simulink model "Vehicle_Control_CodeGen"  (R2024a)
settings: Solver=FixedStepAuto  StartTime=0.0  StopTime=10  RelTol=1e-3  EnableMultiTasking=on
undefined symbols (not defined in the file or in its folder): CAN, DiscIntNeverNeededParam, FD, Ion, Lithium
libraries: stmutilitieslib x28, simulink x21, stm32blockslib x10, canfdmsglib x6, dspstat3 x6, slpidlib x3, spsBatteryLib x2, spsControlledCurrentSourceLib x2, spsVoltageMeasurementLib x2, spspowerguiLib x2, stm32h7xxblockslib x2
(part 1 of 3)
settings Model: STM32="{\"FDCANWrite\":[{\"ID\":\"Vehicle_Control_CodeGen:2627\"},{\"ID\":\"Vehicle_Control_CodeGen:2628\"},{\"ID\":\"Vehicle_Control_CodeGen:2945\"},{\"ID\":\"Vehicle_Control_CodeGen:2946\"},{\"ID\":\"Vehicle_Control_CodeGen:2660\"},{\"ID\":\"Vehicle_Control_CodeGen:2661\"},{\"ID\":\"Vehicle_Control_CodeGen:3556\"},{\"ID\":\"Vehicle_Control_CodeGen:3558\"}],\"FDCANRead\":[{\"ID\":\"Vehicle_Control_CodeGen:2697\"},{\"ID\":\"Vehicle_Control_CodeGen:2816\"}],\"HardwareInterrupt\":[{\"ID\":\"Vehicle_Control_CodeGen:2909\"},{\"ID\":\"Vehicle_Control_CodeGen:2910\"}]}"  Creator=ezeki  LastModifiedBy=ezeki
settings SolverCC: PositivePriorityOrder=on  AutoInsertRateTranBlk=on
settings OptimizationCC: EnhancedBackFolding=on  PassReuseOutputArgsAs=Individual arguments  ZeroExternalMemoryAtStartup=off  ZeroInternalMemoryAtStartup=off  MaxStackSize=512  OptimizeBlockOrder=speed  DifferentSizesBufferReuse=on  OptimizationCustomize=off  EfficientTunableParamExpr=on
settings DebuggingCC: MultiTaskDSMMsg=none  ParameterTunabilityLossMsg=error
settings HardwareCC: ProdBitPerPointer=32  ProdBitPerSizeT=32  ProdBitPerPtrDiffT=32  ProdLargestAtomicInteger=Long  ProdLargestAtomicFloat=Double  ProdWordSize=32  ProdLongLongMode=on  ProdHWDeviceType=ARM Compatible->ARM Cortex-M
settings SFSimCC: MATLABDynamicMemAlloc=off
settings RTWCC: Description=Embedded Coder  SystemTargetFile=ert.tlc  HardwareBoard=STM32H7xx Based (Single-core)  TLCOptions="-aInlineSetEventsForThisBaseRateFcn=TLC_FALSE -aSuppressMultiTaskScheduler=TLC_FALSE  -aRateBasedStepFcn=0"  TemplateMakefile=ert_default_tmf  Toolchain=GNU Tools for ARM Embedded Processors
settings CodeAppCC: ForceParamTrailComments=on  IgnoreCustomStorageClasses=off  OperatorAnnotations=on  SimulinkDataObjDesc=on  SFDataObjDesc=on  InsertBlockDesc=on
settings ERTTargetCC: TargetLangStandard=C99 (ISO)  CodeReplacementLibrary=ARM Cortex-M  ExtModeTransport=3  ExtModeStaticAlloc=on  ExtModeStaticAllocSize=2048  ExtModeMexFile=ext_xcp  ExtModeIntrfLevel=Level2 - Open

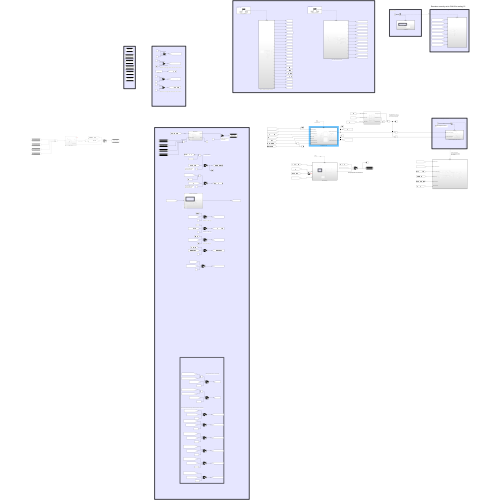
[thumbnail: Simulink's stored preview of the top-level diagram]
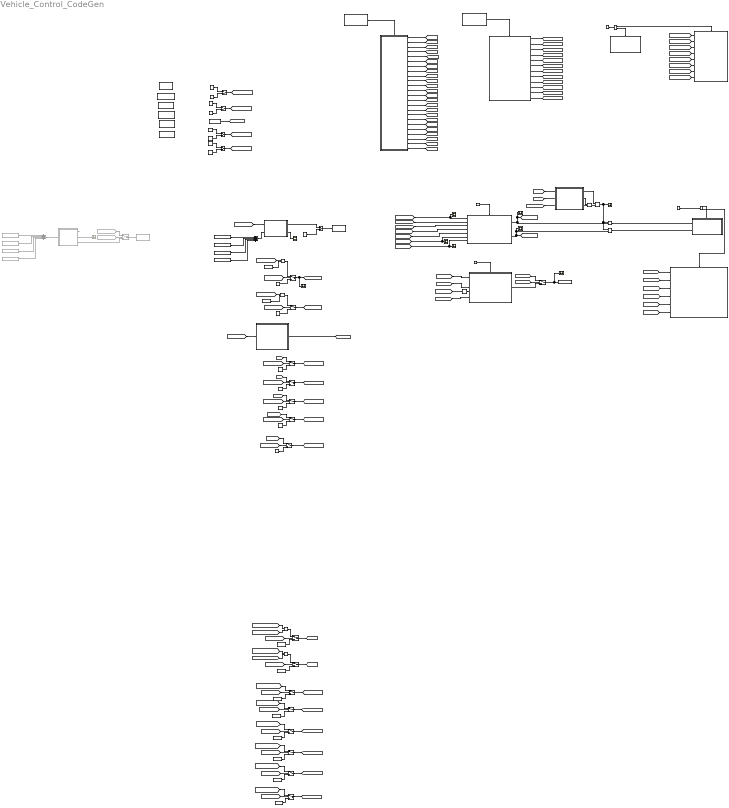
== system Vehicle_Control_CodeGen ==
  note: Because of the expected amount of acceleration between function call this function is also set to run at 50Hz.
  note: Derating values a scalers and are in the the magnitude of 0-1. The can be multiplied by with the requested power to scale them appropriatly.
  note: Takes the greater of the two for use in derating.
  note: Handy to test Can outputs. A constant can be put in to test transmission
  note: Greater then 5 enables regen
  note: Converts RPM to Rad/s
  note: PID Loop runs allot faster to minimise overshoot. Messages are sent at a slower rate.
  note: Remeber currently set to CAN 2 for testing !!!!
  note: Receiving Can messages from CAN 1 (front of vehicle) and Can 2 (inverters)
  note: These can also be used to test code gen. Shows that varibles are transmitting.
  note: Global Defines
  note: Set Max time to 2154 Length of dat set used for power control for endurance
  note: This Constant Can be changed to varible at a latter date for data playback/simulation
  note: All Global Varibles
  note: Simulation Varible Setup
  note: This can be configured for either endurance (Power Forcasting Used) Or other events (fixed power limit)
  note: Set to 500 Hz call
  note: This Constant Can be changed to varible at a latter date for data playback/simulation
  note: Set Max time to 2154 Length of dat set used for power control for endurance
  note: CAN 1 information from pedal box and dash.
  note: Inverter Can Setup
  note: CAN 2 Receive Data From Inverters
  note: Forwarding Messages From the Inverters to Data Logger
  note: Example On How to send Messages to Inverters
  note: Greater then 5 enables regen
  note: Less then 90 enables regen
  10 HZ Send1 : Subsystem  TreatAsAtomicUnit=on
  50 HZ Send Torque Requests to Inverters : Subsystem  TreatAsAtomicUnit=on
  Add : Sum  Commented=on  Inputs=++++
  Add1 : Sum  Inputs=++++
  Battery Model : Subsystem  Commented=on
  Constant{,5,14,24} (4 alike) : Constant
  Constant{1,6,8,15,25} (5 alike) : Constant  Value=0
  Constant{2,7,10..13} (6 alike) : Constant  Value=25000
  Constant16 : Constant  Value=0.10472
  Constant17 : Constant  Value=0.10472
  Constant18 : Constant  Value=6
  Constant19 : Constant  Value=85
  Constant20 : Constant  Value=580
  Constant21 : Constant  Value=20
  Constant22 : Constant  Value=40
  Constant23 : Constant  Value=60
  Constant3 : Constant  Value=10
  Constant4 : Constant  Value=10
  Constant9 : Constant  Value=6
  Data Store Memory : DataStoreMemory  DataStoreName=Battery_Voltage  WriteAfterWriteMsg=warning  ShowAdditionalParam=off
  Data Store Memory1 : DataStoreMemory  DataStoreName=Right_Sim_Discharge_Current  WriteAfterWriteMsg=warning  ShowAdditionalParam=off
  Data Store Memory2 : DataStoreMemory  DataStoreName=Right_Sim_Regen_Current  WriteAfterWriteMsg=warning  ShowAdditionalParam=off
  Data Store Memory3 : DataStoreMemory  DataStoreName=Left_Sim_Discharge_Current  WriteAfterWriteMsg=warning  ShowAdditionalParam=off
  Data Store Memory4 : DataStoreMemory  DataStoreName=Left_Sim_Regen_Current  WriteAfterWriteMsg=warning  ShowAdditionalParam=off
  Data Store Memory5 : DataStoreMemory  DataStoreName=Global_Power_Limit  WriteAfterWriteMsg=warning  ShowAdditionalParam=off
  Data Store Read : DataStoreRead  Commented=on  DataStoreName=Left_Sim_Discharge_Current  IndexOptions=Index vector (dialog)  Indices=1  OutputSizes=1
  Data Store Read1 : DataStoreRead  Commented=on  DataStoreName=Left_Sim_Regen_Current  IndexOptions=Index vector (dialog)  Indices=1  OutputSizes=1
  Data Store Read2 : DataStoreRead  Commented=on  DataStoreName=Right_Sim_Discharge_Current  IndexOptions=Index vector (dialog)  Indices=1  OutputSizes=1
  Data Store Read3 : DataStoreRead  Commented=on  DataStoreName=Right_Sim_Regen_Current  IndexOptions=Index vector (dialog)  Indices=1  OutputSizes=1
  Data Store Read4 : DataStoreRead  DataStoreName=Left_Sim_Discharge_Current  IndexOptions=Index vector (dialog)  Indices=1  OutputSizes=1
  Data Store Read5 : DataStoreRead  DataStoreName=Left_Sim_Regen_Current  IndexOptions=Index vector (dialog)  Indices=1  OutputSizes=1
  Data Store Read6 : DataStoreRead  DataStoreName=Right_Sim_Discharge_Current  IndexOptions=Index vector (dialog)  Indices=1  OutputSizes=1
  Data Store Read7 : DataStoreRead  DataStoreName=Right_Sim_Regen_Current  IndexOptions=Index vector (dialog)  Indices=1  OutputSizes=1
  Data Store Write : DataStoreWrite  Commented=on  DataStoreName=Battery_Voltage  IndexOptions=Index vector (dialog)  Indices=1  OutputSizes=1
  Data Store Write1 : DataStoreWrite  DataStoreName=Global_Power_Limit  IndexOptions=Index vector (dialog)  Indices=1  OutputSizes=1
  Data Store Write2 : DataStoreWrite  DataStoreName=Battery_Voltage  IndexOptions=Index vector (dialog)  Indices=1  OutputSizes=1
  From7 : From  Commented=on  GotoTag=Simulation_Enable
  From8 : From  Commented=on  GotoTag=CAN_Battery_Voltage
  Function-Call Generator : simulink/Ports & Subsystems/Function-Call Generator  sample_time=0.002  numberOfIterations=1  DisallowWideOutput=off
  Function-Call Generator1 : simulink/Ports & Subsystems/Function-Call Generator  sample_time=0.01  numberOfIterations=1  DisallowWideOutput=off
  Function-Call Generator2 : simulink/Ports & Subsystems/Function-Call Generator  sample_time=0.02  numberOfIterations=1  DisallowWideOutput=off
  Function-Call Generator4 : simulink/Ports & Subsystems/Function-Call Generator  sample_time=0.2  numberOfIterations=1  DisallowWideOutput=off
  Function-Call Split : FunctionCallSplit  IconShape=distinctive  NumOutputPorts=2  OutputPortLayout=default
  Function-Call Split1 : FunctionCallSplit  IconShape=distinctive  NumOutputPorts=2
  Function-Call Subsystem : Subsystem  TreatAsAtomicUnit=on
  Function-Call Subsystem1 : Subsystem  TreatAsAtomicUnit=on
  Hardware Interrupt1 : stm32h7xxblockslib/Hardware Interrupt  ISRGroup=Controller Area Network Flexible Data-Rate (FDCAN)  ISRName=FDCAN2_IT0_IRQHandler  ISRNumber=35  EventsList={ 'off', 'FDCAN2 HPME', '1'; 'off', 'FDCAN2 DRXE', '2'; 'on', 'FDCAN2 RF0NE', '3'; 'off', 'FDCAN2 RF0F', '4'; 'off', 'FDCAN2 RF0L', '5'; 'off', 'FDCAN2 RF0W', '6'; 'off', 'FDCAN2 RF1NE', '7'; 'off', 'FDCAN2 RF1F', '8'; 'off', 'FDCAN2 RF1L', '9'; 'off', 'FDCAN2 RF1W', '10'; 'off', 'FDCAN2 TC', '11'; 'off', 'FDCAN2 TCF', '12'; 'off', 'FDCAN2 TFE', '13'; 'off', 'FDCAN2 TEFN', '14'; 'off', 'FDCAN2 TEFL', '15'; 'off', 'FDCAN2 TEFF', '16'; 'off', 'FDCAN2 TEFW', '17'; 'off', 'FDCAN2 TSW', '18'; 'off', 'FDCAN2 MRAF', '19'; 'off', 'FDCAN2 TOO', '20'; 'off', 'FDCAN2 ELO', '21'; 'off', 'FDCAN2 EP', '22'; 'off', 'FDCAN2 EW', '23'; 'off', 'FDCAN2 BO', '24'; 'off', 'FDCAN2 WDI', '25'; 'off', 'FDCAN2 PEA', '26'; 'off', 'FDCAN2 PED', '27'; 'off', 'FDCAN2 ARA', '28'; 'off', 'Custom event', '29' }  SelectedEvents={'FDCAN2 RF0NE'}  TaskPriority=29  DisablePreemption=off  ClearInterruptFlagsAtEndOfEvent=off  InterruptDefinitionFile=$(TARGET_ROOT)/registry/interrupts/STM32F4xxBased_interrupts.xml  HardwareBoard=STM32H7xx Based  EnableSimPort=off
  Hardware Interrupt3 : stm32h7xxblockslib/Hardware Interrupt  ISRGroup=Controller Area Network Flexible Data-Rate (FDCAN)  ISRName=FDCAN1_IT0_IRQHandler  ISRNumber=34  EventsList={ 'off', 'FDCAN1 HPME', '1'; 'off', 'FDCAN1 DRXE', '2'; 'on', 'FDCAN1 RF0NE', '3'; 'off', 'FDCAN1 RF0F', '4'; 'off', 'FDCAN1 RF0L', '5'; 'off', 'FDCAN1 RF0W', '6'; 'off', 'FDCAN1 RF1NE', '7'; 'off', 'FDCAN1 RF1F', '8'; 'off', 'FDCAN1 RF1L', '9'; 'off', 'FDCAN1 RF1W', '10'; 'off', 'FDCAN1 TC', '11'; 'off', 'FDCAN1 TCF', '12'; 'off', 'FDCAN1 TFE', '13'; 'off', 'FDCAN1 TEFN', '14'; 'off', 'FDCAN1 TEFL', '15'; 'off', 'FDCAN1 TEFF', '16'; 'off', 'FDCAN1 TEFW', '17'; 'off', 'FDCAN1 TSW', '18'; 'off', 'FDCAN1 MRAF', '19'; 'off', 'FDCAN1 TOO', '20'; 'off', 'FDCAN1 ELO', '21'; 'off', 'FDCAN1 EP', '22'; 'off', 'FDCAN1 EW', '23'; 'off', 'FDCAN1 BO', '24'; 'off', 'FDCAN1 WDI', '25'; 'off', 'FDCAN1 PEA', '26'; 'off', 'FDCAN1 PED', '27'; 'off', 'FDCAN1 ARA', '28'; 'off', 'Custom event', '29' }  SelectedEvents={'FDCAN1 RF0NE'}  TaskPriority=30  DisablePreemption=off  ClearInterruptFlagsAtEndOfEvent=off  InterruptDefinitionFile=$(TARGET_ROOT)/registry/interrupts/STM32F4xxBased_interrupts.xml  HardwareBoard=STM32H7xx Based  EnableSimPort=off
  Manual Switch{,1..2,4} (4 alike) : ManualSwitch  CurrentSetting=0
  Manual Switch3 : ManualSwitch
  Max : MinMax  Function=max  Inputs=2
  Max1 : MinMax  Function=max  Inputs=2
  Power Forcasting : Subsystem  TreatAsAtomicUnit=on
  Power Limit : Constant  Value=50000
  Product{,1..5} (6 alike) : Product
  Rate Transition : RateTransition
  Scope{,1..3,5..9} (9 alike) : Scope
  Scope4 : Scope  Commented=on
  Subsystem : Subsystem
  Switch : Switch  Commented=on  Criteria=u2 > Threshold  Threshold=0.5  SaturateOnIntegerOverflow=off  InputSameDT=off
  Switch{1..16} (16 alike) : Switch  Criteria=u2 > Threshold  Threshold=0.5  SaturateOnIntegerOverflow=off  InputSameDT=off
  Throttle/Regen Control : Subsystem  TreatAsAtomicUnit=on
  Triggered Subsystem : Subsystem  TreatAsAtomicUnit=on
  Triggered Subsystem1 : Subsystem  TreatAsAtomicUnit=on
  Variant Subsystem : Subsystem  Variant=on  VariantControlMode=sim codegen switching
  Variant Subsystem1 : Subsystem  Variant=on  VariantControlMode=sim codegen switching
  wires:
  [Throttle_Percent_Global] -> Scope6/1, Throttle/Regen Control/1(Throttle Percentage)
  Manual Switch/1 -> [Simulation_Enable]
  Constant1/1 -> Manual Switch/2  "Simulate"
  Constant/1 -> Manual Switch/1  "Code Gen"
  Function-Call Generator/1 -> Throttle/Regen Control/Trigger
  Function-Call Generator1/1 -> Power Forcasting/Trigger  "100Hz"
  Switch3/1 -> Scope3/1, Data Store Write1/1
  Power Forcasting/1(Out1) -> Switch3/3
  Battery Model/3(Batter Voltage) -> Switch/3
  Battery Model/1(m) -> ?
  Add/1 -> Battery Model/1(s)
  Battery Model/2(Out2) -> Scope4/1  "Battery Voltage"
  [Right_Motor_Speed_Rads] -> Scope8/1, Throttle/Regen Control/7(Right Motor Speed (rads))
  [Left_Motor_Speed_Rads] -> Scope7/1, Throttle/Regen Control/6(Left Motor Speed (rads))
  From7/1 -> Switch/2
  From8/1 -> Switch/1
  Data Store Read/1 -> Add/1
  Data Store Read1/1 -> Add/2
  Data Store Read2/1 -> Add/3
  Data Store Read3/1 -> Add/4
  [Simulation_Enable] -> Switch1/2
  Switch1/1 -> Scope2/1, [Left_Motor_Speed_Rads]
  Constant3/1 -> Switch1/3
  Product/1 -> Switch1/1
  Switch2/1 -> [Right_Motor_Speed_Rads]
  [Simulation_Enable] -> Switch2/2
  Constant4/1 -> Switch2/3
  Product1/1 -> Switch2/1
  Constant6/1 -> Manual Switch2/2  "Endurance (Power Forcasting)"
  Manual Switch2/1 -> [PowerLimit_Enable]
  Constant5/1 -> Manual Switch2/1  "Fixed Power Limit"
  [PowerLimit_Enable] -> Switch3/2
  [Fixed_Power_Limit] -> Switch3/1
  Power Limit/1 -> [Fixed_Power_Limit]
  [Right_Wheel_Speed_Ms] -> Power Forcasting/1(In1)
  [Left_Wheel_Speed_Ms] -> Power Forcasting/2(In2)
  [Simulation_Enable] -> Rate Transition/1
  [CAN_SOC] -> Power Forcasting/3(Inport)
  Function-Call Split/2 -> 10 HZ Send1/Trigger
  Function-Call Subsystem1/15(Out15) -> [Brake_Percent]
  Hardware Interrupt1/1 -> Function-Call Subsystem/Trigger
  Function-Call Generator2/1 -> Function-Call Split1/1  "50Hz"
  Function-Call Subsystem1/5(Out5) -> [SCBOTS]
  [LEFT_Inverter_Motor_Voltage] -> Triggered Subsystem/4(In4)
  Function-Call Subsystem/3(Out3) -> [CAN_LEFT_Inverter_Motor_Speed]
  Function-Call Subsystem/9(Out9) -> [CAN_RIGHT_Inverter_Motor_Speed]
  Function-Call Subsystem1/7(Out7) -> [BSEFail]
  Function-Call Subsystem1/6(Out6) -> [APPSFail]
  [Right_Motor_Speed_Rads] -> Triggered Subsystem/6(In6)
  Function-Call Split/1 -> Triggered Subsystem/Trigger  "10Hz"
  [RIGHT_Inverter_Motor_Voltage] -> Triggered Subsystem/8(In8)
  Function-Call Subsystem/1(Out1) -> [CAN_LEFT_Inverter_Bus_Voltage]
  Function-Call Subsystem/6(Out6) -> [CAN_LEFT_Inverter_Motor_Voltage]
  [RIGHT_Inverter_Bus_Voltage] -> Triggered Subsystem/5(In5)
  [Left_Motor_Speed_Rads] -> Triggered Subsystem/2(In2)
  [LEFT_Inverter_Bus_Voltage] -> Triggered Subsystem/1(In1)
  [LEFT_Inverter_Motor_Current] -> Triggered Subsystem/3(In3)
  Function-Call Subsystem/8(Out8) -> [CAN_RIGHT_Inverter_IGBT_temp]
  Function-Call Subsystem/7(Out7) -> [CAN_RIGHT_Inverter_Bus_Voltage]
  Function-Call Subsystem/10(Out10) -> [CAN_RIGHT_Inverter_Motor_Temp]
  Function-Call Subsystem1/1(Out1) -> [Start_Button]
  Function-Call Subsystem1/21(Out21) -> [BMS_SOC]
  Function-Call Subsystem1/11(Out11) -> [SoftwareBSPD]
  Function-Call Subsystem1/18(Out18) -> [WSFR]
  Function-Call Subsystem1/19(Out19) -> [BMS_Current]
  Function-Call Subsystem1/13(Out13) -> [BSEMatch]
  Function-Call Subsystem1/17(Out17) -> [WSFL]
  Function-Call Subsystem1/20(Out20) -> [BMS_Voltage]
  Function-Call Subsystem1/16(Out16) -> [SteeringPercent]
  Function-Call Subsystem1/23(Out23) -> [BMS_Max_CellTemp]
  Function-Call Subsystem1/24(Out24) -> [BMS_Min_CellTemp]
  [RIGHT_Inverter_Motor_Current] -> Triggered Subsystem/7(In7)
  Function-Call Subsystem1/8(Out8) -> [SteeringFail]
  Function-Call Generator4/1 -> Function-Call Split/1  "10Hz"
  Function-Call Subsystem1/22(Out22) -> [BMS_Temprature]
  Function-Call Subsystem/11(Out11) -> [CAN_RIGHT_Inverter_Motor_Current]
  Function-Call Subsystem1/14(Out14) -> [APPS_Percent]
  Function-Call Subsystem1/2(Out2) -> [SCin]
  Function-Call Subsystem/12(Out12) -> [CAN_RIGHT_Inverter_Motor_Voltage]
  Function-Call Subsystem1/9(Out9) -> [APPSMatch]
  Function-Call Subsystem1/3(Out3) -> [SCEstop]
  Function-Call Subsystem1/4(Out4) -> [SCis]
  Hardware Interrupt3/1 -> Function-Call Subsystem1/Trigger
  Function-Call Subsystem/2(Out2) -> [CAN_LEFT_Inverter_IGBT_temp]
  Function-Call Subsystem1/12(Out12) -> [SoftwareError]
  Function-Call Subsystem/4(Out4) -> [CAN_LEFT_Inverter_Motor_Temp]
  Function-Call Subsystem1/10(Out10) -> [BrakesON]
  Function-Call Subsystem/5(Out5) -> [CAN_LEFT_Inverter_Motor_Current]
  Constant2/1 -> Switch5/3
  [CAN_Simulation_Enable] -> Switch5/2
  Switch5/1 -> [LEFT_Inverter_Bus_Voltage]
  [CAN_LEFT_Inverter_Bus_Voltage] -> Switch5/1
  Switch7/1 -> [LEFT_Inverter_Motor_Current]
  Constant7/1 -> Switch7/3
  [CAN_Simulation_Enable] -> Switch7/2
  [CAN_LEFT_Inverter_Motor_Current] -> Switch7/1
  Switch8/1 -> [LEFT_Inverter_Motor_Voltage]
  Constant12/1 -> Switch8/3
  [CAN_Simulation_Enable] -> Switch8/2
  [CAN_LEFT_Inverter_Motor_Voltage] -> Switch8/1
  Switch9/1 -> [RIGHT_Inverter_Bus_Voltage]
  Constant13/1 -> Switch9/3
  [CAN_Simulation_Enable] -> Switch9/2
  [CAN_RIGHT_Inverter_Bus_Voltage] -> Switch9/1
  Switch11/1 -> [RIGHT_Inverter_Motor_Current]
  Constant10/1 -> Switch11/3
  [CAN_Simulation_Enable] -> Switch11/2
  [CAN_RIGHT_Inverter_Motor_Current] -> Switch11/1
  [CAN_Simulation_Enable] -> Switch12/2
  Switch12/1 -> [RIGHT_Inverter_Motor_Voltage]
  Constant11/1 -> Switch12/3
  [CAN_RIGHT_Inverter_Motor_Voltage] -> Switch12/1
  Rate Transition/1 -> ?
  Switch/1 -> Data Store Write/1
  Manual Switch1/1 -> [CAN_Simulation_Enable]
  Constant15/1 -> Manual Switch1/2  "Simulate"
  Constant14/1 -> Manual Switch1/1  "Code Gen"
  [APPS_Percent] -> Variant Subsystem/1(In1)
  [CAN_Battery_Voltage] -> Variant Subsystem1/1(Can Sig)  "CAN Sig"
  Data Store Read5/1 -> Add1/2
  Data Store Read6/1 -> Add1/3
  Add1/1 -> Variant Subsystem1/2(Requested Current)  "Requested Current"
  Data Store Read7/1 -> Add1/4
  Data Store Read4/1 -> Add1/1
  Manual Switch3/1 -> Data Store Write2/1
  Variant Subsystem1/2(Scope) -> Scope5/1
  [CAN_LEFT_Inverter_Motor_Speed] -> Product/1
  Constant16/1 -> Product/2
  Constant17/1 -> Product1/2
  [CAN_RIGHT_Inverter_Motor_Speed] -> Product1/1
  Throttle/Regen Control/1(Right Motor Requested Torque) -> Product2/2, Scope/1, [RightMotor_Torque_Request]
  Throttle/Regen Control/2(Left Motor Requested Torque) -> Scope1/1, Product5/2, [LeftMotor_Torque_Request]
  Variant Subsystem1/1(Batt Out) -> Manual Switch3/1
  Constant20/1 -> Manual Switch3/2
  [WSFR] -> Switch10/1
  [Simulation_Enable] -> Switch10/2
  Switch10/1 -> [Right_Wheel_Speed_Ms]
  Constant9/1 -> Switch10/3
  [Right_Wheel_Speed_Ms] -> Throttle/Regen Control/2(FR Wheel Speed (m/s))
  [Left_Wheel_Speed_Ms] -> Throttle/Regen Control/3(FL Wheel Speed (m/s)1)
  Constant18/1 -> Switch13/3
  [Simulation_Enable] -> Switch13/2
  Switch13/1 -> [Left_Wheel_Speed_Ms]
  [WSFL] -> Switch13/1
  [Simulation_Enable] -> Switch14/2
  Constant19/1 -> Switch14/3
  [BMS_SOC] -> Switch14/1
  Switch14/1 -> [Battery_SOC]
  [Battery_SOC] -> Throttle/Regen Control/5(Battery SOC)
  Switch15/1 -> [Battery_Temprature]
  Constant21/1 -> Switch15/3
  [Simulation_Enable] -> Switch15/2
  [BMS_Temprature] -> Switch15/1
  [Battery_Temprature] -> Throttle/Regen Control/4(Battery Temp)
  Variant Subsystem/1(Out1) -> [Throttle_Percent_Global]
  [MotorTemp] -> Subsystem/2(Motor Temp)  "Motor Temp"
  [Battery_Temprature] -> Subsystem/3(Battery Temp)  "Battery Temp"
  [Inverter_Temp] -> Subsystem/1(IGBT Temp)  "IGBT Temp"
  Product2/1 -> 50 HZ Send Torque Requests to Inverters/1(Right Motor Torque Request)
  Subsystem/3(Derating Constant2) -> Product3/2
  Subsystem/2(Derating Constant1) -> Product3/1
  Product3/1 -> Product4/2
  Subsystem/1(Derating Constant) -> Product4/1
  Product4/1 -> Product5/1, Product2/1, Scope9/1
  Product5/1 -> 50 HZ Send Torque Requests to Inverters/2(Left Motor Torque Request)
  [CAN_LEFT_Inverter_IGBT_temp] -> Max/1
  [CAN_RIGHT_Inverter_IGBT_temp] -> Max/2
  [CAN_LEFT_Inverter_Motor_Temp] -> Max1/1
  [CAN_RIGHT_Inverter_Motor_Temp] -> Max1/2
  Constant22/1 -> Switch6/3
  [CAN_Simulation_Enable] -> Switch6/2
  Switch6/1 -> [Inverter_Temp]
  Max/1 -> Switch6/1
  Constant23/1 -> Switch16/3
  [CAN_Simulation_Enable] -> Switch16/2
  Switch16/1 -> [MotorTemp]
  Max1/1 -> Switch16/1
  Function-Call Split1/1 -> 50 HZ Send Torque Requests to Inverters/Trigger
  Function-Call Split1/2 -> Triggered Subsystem1/Trigger
  [Left_Wheel_Speed_Ms] -> Triggered Subsystem1/2(Front Left Wheel Speed)
  [Right_Wheel_Speed_Ms] -> Triggered Subsystem1/3(Front Right Wheel Speed)
  [Left_Motor_Speed_Rads] -> Triggered Subsystem1/1(Left Motor Speed)
  [Right_Motor_Speed_Rads] -> Triggered Subsystem1/5(Right Motor Speed)
  Constant8/1 -> Switch4/3
  Switch4/1 -> [Steering_Angle]
  [Simulation_Enable] -> Switch4/2
  [SteeringPercent] -> Switch4/1
  [Steering_Angle] -> Triggered Subsystem1/4(Steering Angle)
  Constant24/1 -> Manual Switch4/1  "Slip Control Enabled"
  Constant25/1 -> Manual Switch4/2  "Slip Control Disabled)"
  Manual Switch4/1 -> [Slip_Control_Enable]
  [Slip_Control_Enable] -> Triggered Subsystem1/6(Slip Control Enable)

== system Vehicle_Control_CodeGen/10 HZ Send1 ==
  note: Messages to the Inverters are only sent twice at startup. This is total of 12 messages.
  function : TriggerPort  TriggerType=function-call  VariantControl=(inherit)
  Constant : Constant
  Constant1 : Constant  Value=0
  Constant2 : Constant
  Constant3 : Constant  Value=12
  Enabled Subsystem : Subsystem  TreatAsAtomicUnit=on
  GreaterThan : RelationalOperator  Operator=>  OutDataTypeStr=boolean  RndMeth=Simplest  InputSameDT=off
  Scope : Scope
  Scope1 : Scope
  Sum : Sum  Inputs=|++
  Switch : Switch  Criteria=u2 > Threshold  SaturateOnIntegerOverflow=off  InputSameDT=off
  Unit Delay : UnitDelay  SampleTime=-1  HasFrameUpgradeWarning=on
  wires:
  Constant/1 -> Sum/2
  Unit Delay/1 -> Sum/1
  Sum/1 -> GreaterThan/1, Unit Delay/1
  Constant1/1 -> Switch/1
  Constant2/1 -> Switch/3
  Constant3/1 -> GreaterThan/2
  GreaterThan/1 -> Scope1/1, Switch/2
  Switch/1 -> Enabled Subsystem/Enable, Scope/1

== system Vehicle_Control_CodeGen/50 HZ Send Torque Requests to Inverters ==
  note: This is the Register Address which torque is sent to
  note: Byte reversal is used so that the low byte appears to the left of the high byte
  note: This is the Register Address which torque is sent to
  note: Byte reversal is used so that the low byte appears to the left of the high byte
  note: Torque Request To Right Inverter
  note: Torque Request To Left Inverter
  Right Motor Torque Request : Inport
  Left Motor Torque Request : Inport  Port=2
  function : TriggerPort  TriggerType=function-call  VariantControl=(inherit)
  Byte Pack : stmutilitieslib/Byte Pack  datatypes={'int16'}  byteAlign=1  blockPlatform=stm32f4discovery
  Byte Pack1 : stmutilitieslib/Byte Pack  datatypes={'int16'}  byteAlign=1  blockPlatform=stm32f4discovery
  Byte Reversal : stmutilitieslib/Byte Reversal  numInp=1  blockPlatform=stm32f4discovery
  Byte Reversal1 : stmutilitieslib/Byte Reversal  numInp=1  blockPlatform=stm32f4discovery
  Constant1 : Constant  Value=144
  Constant3 : Constant  Value=144
  Data Type Conversion : DataTypeConversion  OutDataTypeStr=int16  SaturateOnIntegerOverflow=off  RndMeth=Floor
  Data Type Conversion1 : DataTypeConversion  OutDataTypeStr=uint8  SaturateOnIntegerOverflow=off  RndMeth=Floor
  Data Type Conversion2 : DataTypeConversion  OutDataTypeStr=int16  SaturateOnIntegerOverflow=off  RndMeth=Floor
  Data Type Conversion3 : DataTypeConversion  OutDataTypeStr=uint8  SaturateOnIntegerOverflow=off  RndMeth=Floor
  FDCAN Write1 : stm32blockslib/FDCAN Write  FDCANModule=FDCAN2  BlockMode=Transmit  OperationReadMode=Data  OperationWriteMode=Data  ReadSource=FIFO 0  BufferNumber=0  OutputTypeReadMode=Unpacked  DataFormatWriteMode=Raw data  CANFrameType=CAN  IdentifierTypeVia=Dialog  IdentifierType=Standard (11-bit identifier)  IdentifierVia=Dialog  Identifier=529  DataLengthVia=Dialog  DataLength=3  OutputIdType=off  IsBitRateSwitchingEnabled=off  TransmitRemoteFrame=off  OutputFrameType=off  OutputBRS=off  OutputRemoteFrame=off  OutputTxFifoLevel=off  OutputRxFifoLevel=off  OutputStatus=off  Timeout=1  SampleTime=-1
      settings: LibrarySourceBlock=stm32l5xxblockslib/FDCAN Write
  FDCAN Write3 : stm32blockslib/FDCAN Write  FDCANModule=FDCAN2  BlockMode=Transmit  OperationReadMode=Data  OperationWriteMode=Data  ReadSource=FIFO 0  BufferNumber=0  OutputTypeReadMode=Unpacked  DataFormatWriteMode=Raw data  CANFrameType=CAN  IdentifierTypeVia=Dialog  IdentifierType=Standard (11-bit identifier)  IdentifierVia=Dialog  Identifier=528  DataLengthVia=Dialog  DataLength=3  OutputIdType=off  IsBitRateSwitchingEnabled=off  TransmitRemoteFrame=off  OutputFrameType=off  OutputBRS=off  OutputRemoteFrame=off  OutputTxFifoLevel=off  OutputRxFifoLevel=off  OutputStatus=off  Timeout=1  SampleTime=-1
      settings: LibrarySourceBlock=stm32l5xxblockslib/FDCAN Write
  Vector Concatenate : Concatenate
  Vector Concatenate1 : Concatenate
  wires:
  Right Motor Torque Request/1 -> Data Type Conversion/1
  Data Type Conversion/1 -> Byte Reversal/1
  Byte Pack/1 -> Vector Concatenate/2
  Byte Reversal/1 -> Byte Pack/1
  Vector Concatenate/1 -> FDCAN Write1/1
  Constant1/1 -> Data Type Conversion1/1
  Data Type Conversion1/1 -> Vector Concatenate/1
  Data Type Conversion2/1 -> Byte Reversal1/1
  Vector Concatenate1/1 -> FDCAN Write3/1
  Byte Pack1/1 -> Vector Concatenate1/2
  Left Motor Torque Request/1 -> Data Type Conversion2/1
  Data Type Conversion3/1 -> Vector Concatenate1/1
  Byte Reversal1/1 -> Byte Pack1/1
  Constant3/1 -> Data Type Conversion3/1

== system Vehicle_Control_CodeGen/Battery Model ==
  note: Delay increased to 3 x 0.01 second to test robustness. This is to simulate the delay of having voltage measurments sent to the VCU
  note: Battery Model is from SIM SCAPE Tool box. Uses a constant current drive to take the current request from controller and apply load to the battery
  s : Inport
  Battery1 : spsBatteryLib/Battery  BatType=Lithium-Ion  ShowTempParam=off  ThermalPreset=no  ShowAgeParam=off  NomV=532.8  NomQ=1152  SOC=85  Batt_Tr=5  PresetModel=on  MaxQ=1152  MinV=399.6  FullV=620.1723  Dis_rate=500.8696  R=0.004625  Normal_OP=1041.8087  expZone="[575.6296      56.59826]"  current=[6.5 13 32.5]  Units=Time  Tci=20  NomT=20  T2=-30  MaxQ2=4.8  FullV2=7.1  Normal_OP2=5.655  expZone2="[6.58           1]"  Rca=0.6  ti=2000  Dp=0  Neq0=0  Tsim=1e6  Ta1=25  Qeol=5.4*0.9  Reol=0.013333*1.2  Char_age=[2.3478, 3]  Dis_age=[2.3478, 10]  N1=1500  N2=10500  N3=1000  N4=1400  Ta2=45  N5=950
  Controlled Current Source1 : spsControlledCurrentSourceLib/Controlled Current Source  Initialize=on  Source_Type=AC  Amplitude=0  Phase=0  Frequency=0  Measurements=None
  Delay2 : Delay  DelayLength=5  InitialCondition=580
  Scope5 : Scope
  Voltage Measurement1 : spsVoltageMeasurementLib/Voltage Measurement  PhasorSimulation=off  OutputType=Complex  PSBequivalent=0
  powergui1 : spspowerguiLib/powergui  Priority=1  SimulationMode=Discrete  SampleTime=0.001  frequency=60  Iterations=50  frequencyindice=0  Pbase=100e6  ErrMax=1e-4  UnitsV=kV  UnitsW=MW  buscounter=0  FunctionMessages=off  echomessages=off  EnableUseOfTLC=off  CurrentSourceSwitches=off  DisableSnubberDevices=off  DisableRonSwitches=off  DisableVfSwitches=off  DisplayEquations=off  AutomaticDiscreteSolvers=off  SolverType=Tustin/Backward Euler (TBE)  Interpol=off  ExternalGateDelay=off  methode=off  Ts=100  x0status=blocks  SPID=on  SwTol=0  HookPort=off  NonlinearTolerance=1e-4  nMaxIteration=100  ContinueOnMaxIteration=off  RestoreLinks=warning  ResistiveCurrentMeasurement=off  Frange=[0:2:500]  Ylog=off  Xlog=on  ShowGrid=off  save=off  variable=ZData  structure=0  ZoomFFT=off  StartTime=0.0  cycles=1  DisplayStyle=1  fundamental=60  FreqAxis=off  MaxFrequency=1000  frequencyindicesteady=1  RmsSteady=1  display=off
  m : Outport
  Out2 : Outport  Port=2
  Batter Voltage : Outport  Port=3
  wires:
  Voltage Measurement1/1 -> Delay2/1, Out2/1, Scope5/1  "BUS Voltage"
  s/1 -> Controlled Current Source1/1
  Delay2/1 -> Batter Voltage/1  "Batter Voltage"
  Battery1/1 -> m/1
  connections:
  Voltage Measurement1/LConn1 -- Controlled Current Source1/RConn1 -- Battery1/LConn1
  Battery1/LConn2 -- Voltage Measurement1/LConn2 -- Controlled Current Source1/LConn1

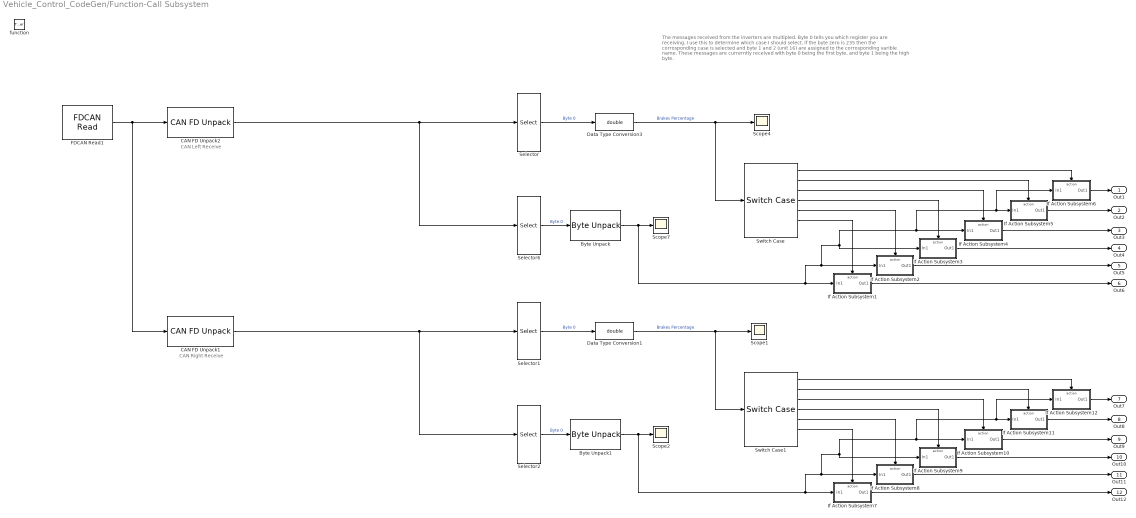
== system Vehicle_Control_CodeGen/Function-Call Subsystem ==
  note: The messages received from the inverters are multipled. Byte 0 tells you which register you are receiving. I use this to determine which case I should select. if the byte zero is 235 then the corrosponding case is selected and byte 1 and 2 (unit 16) are assigned to the corrosponding varible name. These messages are currerntly received with byte 0 being the first byte, and byte 1 being the high byte.
  note: CAN Left Receive
  note: CAN Right Receive
  function : TriggerPort  TriggerType=function-call  VariantControl=(inherit)
  Byte Unpack : stmutilitieslib/Byte Unpack  dimensions={[1]}  datatypes={'uint16'}  byteAlign=1  blockPlatform=stm32f4discovery
  Byte Unpack1 : stmutilitieslib/Byte Unpack  dimensions={[1]}  datatypes={'uint16'}  byteAlign=1  blockPlatform=stm32f4discovery
  CAN FD Unpack1 : canfdmsglib/CAN FD Unpack  MsgList=(none)  MsgName=Msg  ProtocolMode=CAN  MsgIDType=Standard (11-bit identifier)  MsgIdentifier=401  MsgLength=3  SignalInfo={}  IDPort=off  TimestampPort=off  ErrorPort=off  RemotePort=off  LengthPort=off  StatusPort=off  BRSPort=off  ESIPort=off  DLCPort=off  ApplyMinMax=off
      settings: LibrarySourceBlock=stmutilitieslib/CAN FD Unpack  DataFormat=raw data
  CAN FD Unpack2 : canfdmsglib/CAN FD Unpack  MsgList=(none)  MsgName=Msg  ProtocolMode=CAN  MsgIDType=Standard (11-bit identifier)  MsgIdentifier=400  MsgLength=3  SignalInfo={}  IDPort=off  TimestampPort=off  ErrorPort=off  RemotePort=off  LengthPort=off  StatusPort=off  BRSPort=off  ESIPort=off  DLCPort=off  ApplyMinMax=off
      settings: LibrarySourceBlock=stmutilitieslib/CAN FD Unpack  DataFormat=raw data
  Data Type Conversion1 : DataTypeConversion  OutDataTypeStr=double  SaturateOnIntegerOverflow=off  RndMeth=Floor
  Data Type Conversion3 : DataTypeConversion  OutDataTypeStr=double  SaturateOnIntegerOverflow=off  RndMeth=Floor
  FDCAN Read1 : stm32blockslib/FDCAN Read  FDCANModule=FDCAN2  BlockMode=Receive  OperationReadMode=Data  OperationWriteMode=Data  ReadSource=FIFO 0  BufferNumber=0  OutputTypeReadMode=Packed  DataFormatWriteMode=Raw data  CANFrameType=CAN-FD  IdentifierTypeVia=Dialog  IdentifierType=Standard (11-bit identifier)  IdentifierVia=Inport  Identifier=100  DataLengthVia=Inport  DataLength=64  OutputIdType=off  IsBitRateSwitchingEnabled=off  TransmitRemoteFrame=off  OutputFrameType=off  OutputBRS=off  OutputRemoteFrame=off  OutputTxFifoLevel=off  OutputRxFifoLevel=off  OutputStatus=off  Timeout=0.001  SampleTime=-1
      settings: LibrarySourceBlock=stm32l5xxblockslib/FDCAN Read
  If Action Subsystem1 : Subsystem  TreatAsAtomicUnit=on
  If Action Subsystem10 : Subsystem  TreatAsAtomicUnit=on
  If Action Subsystem11 : Subsystem  TreatAsAtomicUnit=on
  If Action Subsystem12 : Subsystem  TreatAsAtomicUnit=on
  If Action Subsystem2 : Subsystem  TreatAsAtomicUnit=on
  If Action Subsystem3 : Subsystem  TreatAsAtomicUnit=on
  If Action Subsystem4 : Subsystem  TreatAsAtomicUnit=on
  If Action Subsystem5 : Subsystem  TreatAsAtomicUnit=on
  If Action Subsystem6 : Subsystem  TreatAsAtomicUnit=on
  If Action Subsystem7 : Subsystem  TreatAsAtomicUnit=on
  If Action Subsystem8 : Subsystem  TreatAsAtomicUnit=on
  If Action Subsystem9 : Subsystem  TreatAsAtomicUnit=on
  Scope{1..2,4,7} (4 alike) : Scope
  Selector : Selector  InputPortWidth=3  IndexOptions=Index vector (dialog)  Indices=[1 ]  OutputSizes=1
  Selector1 : Selector  InputPortWidth=3  IndexOptions=Index vector (dialog)  Indices=[1 ]  OutputSizes=1
  Selector2 : Selector  InputPortWidth=3  IndexOptions=Index vector (dialog)  Indices=[2 3 ]  OutputSizes=1
  Selector6 : Selector  InputPortWidth=3  IndexOptions=Index vector (dialog)  Indices=[2 3 ]  OutputSizes=1
  Switch Case : SwitchCase  CaseConditions={235, 74, 168, 73, 95, 138}
  Switch Case1 : SwitchCase  CaseConditions={235, 74, 168, 73, 95, 138}
  Out1 : Outport
  Out2 : Outport  Port=2
  Out3 : Outport  Port=3
  Out4 : Outport  Port=4
  Out5 : Outport  Port=5
  Out6 : Outport  Port=6
  Out7 : Outport  Port=7
  Out8 : Outport  Port=8
  Out9 : Outport  Port=9
  Out10 : Outport  Port=10
  Out11 : Outport  Port=11
  Out12 : Outport  Port=12
  wires:
  FDCAN Read1/1 -> CAN FD Unpack1/1, CAN FD Unpack2/1
  CAN FD Unpack2/1 -> Selector6/1, Selector/1
  Selector/1 -> Data Type Conversion3/1  "Byte 0"
  Data Type Conversion3/1 -> Scope4/1, Switch Case/1  "Brakes Percentage"
  Byte Unpack/1 -> If Action Subsystem6/1(In1), If Action Subsystem5/1(In1), If Action Subsystem4/1(In1), If Action Subsystem3/1(In1), If Action Subsystem2/1(In1), If Action Subsystem1/1(In1), Scope7/1
  Selector6/1 -> Byte Unpack/1  "Byte 0"
  Switch Case/6 -> If Action Subsystem1/Action
  If Action Subsystem1/1(Out1) -> Out6/1
  Switch Case/5 -> If Action Subsystem2/Action
  Switch Case/4 -> If Action Subsystem3/Action
  Switch Case/3 -> If Action Subsystem4/Action
  Switch Case/2 -> If Action Subsystem5/Action
  Switch Case/1 -> If Action Subsystem6/Action
  If Action Subsystem6/1(Out1) -> Out1/1
  If Action Subsystem5/1(Out1) -> Out2/1
  If Action Subsystem4/1(Out1) -> Out3/1
  If Action Subsystem2/1(Out1) -> Out5/1
  If Action Subsystem3/1(Out1) -> Out4/1
  Selector2/1 -> Byte Unpack1/1  "Byte 0"
  Switch Case1/6 -> If Action Subsystem7/Action
  Byte Unpack1/1 -> If Action Subsystem12/1(In1), If Action Subsystem11/1(In1), If Action Subsystem10/1(In1), If Action Subsystem9/1(In1), If Action Subsystem8/1(In1), If Action Subsystem7/1(In1), Scope2/1
  Data Type Conversion1/1 -> Scope1/1, Switch Case1/1  "Brakes Percentage"
  If Action Subsystem10/1(Out1) -> Out9/1
  Switch Case1/2 -> If Action Subsystem11/Action
  Switch Case1/3 -> If Action Subsystem10/Action
  If Action Subsystem7/1(Out1) -> Out12/1
  Selector1/1 -> Data Type Conversion1/1  "Byte 0"
  If Action Subsystem11/1(Out1) -> Out8/1
  If Action Subsystem9/1(Out1) -> Out10/1
  If Action Subsystem12/1(Out1) -> Out7/1
  Switch Case1/5 -> If Action Subsystem8/Action
  Switch Case1/4 -> If Action Subsystem9/Action
  If Action Subsystem8/1(Out1) -> Out11/1
  Switch Case1/1 -> If Action Subsystem12/Action
  CAN FD Unpack1/1 -> Selector2/1, Selector1/1

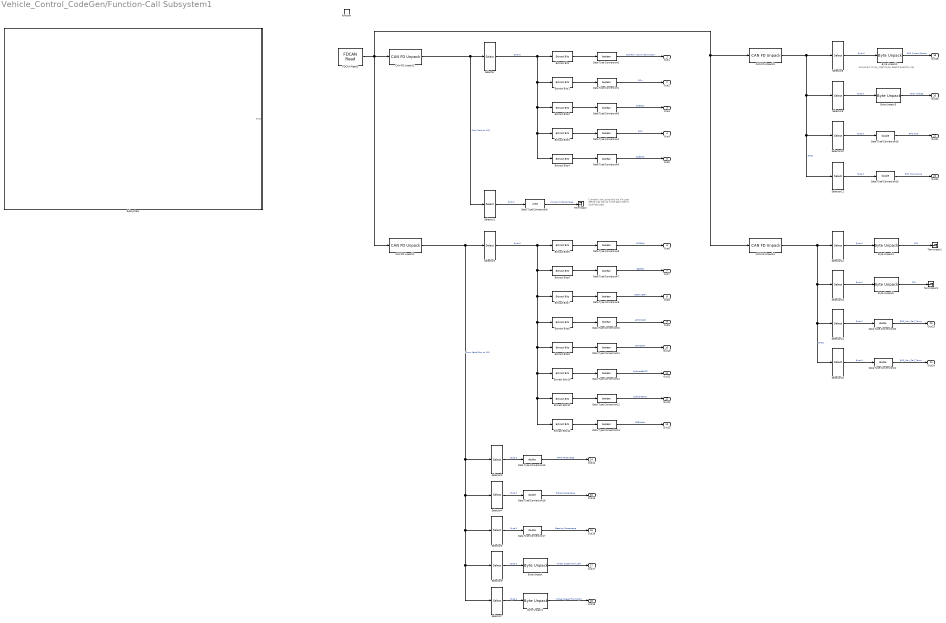
== system Vehicle_Control_CodeGen/Function-Call Subsystem1 ==
  note: Assume it is low_hight byte, doesnt explicity say
  note: Currently not using this but if a user define was set up in the dash then it could be used.
  function : TriggerPort  TriggerType=function-call  VariantControl=(inherit)
  Byte Unpack{,1..5} (6 alike) : stmutilitieslib/Byte Unpack  dimensions={[1]}  datatypes={'uint16'}  byteAlign=1  blockPlatform=stm32f4discovery
  CAN FD Unpack1 : canfdmsglib/CAN FD Unpack  MsgList=(none)  MsgName=Msg  ProtocolMode=CAN  MsgIDType=Standard (11-bit identifier)  MsgIdentifier=1  MsgLength=8  SignalInfo={}  IDPort=off  TimestampPort=off  ErrorPort=off  RemotePort=off  LengthPort=off  StatusPort=off  BRSPort=off  ESIPort=off  DLCPort=off  ApplyMinMax=off
      settings: LibrarySourceBlock=stmutilitieslib/CAN FD Unpack  DataFormat=raw data
  CAN FD Unpack2 : canfdmsglib/CAN FD Unpack  MsgList=(none)  MsgName=Msg  ProtocolMode=CAN  MsgIDType=Standard (11-bit identifier)  MsgIdentifier=2  MsgLength=8  SignalInfo={}  IDPort=off  TimestampPort=off  ErrorPort=off  RemotePort=off  LengthPort=off  StatusPort=off  BRSPort=off  ESIPort=off  DLCPort=off  ApplyMinMax=off
      settings: LibrarySourceBlock=stmutilitieslib/CAN FD Unpack  DataFormat=raw data
  CAN FD Unpack3 : canfdmsglib/CAN FD Unpack  MsgList=(none)  MsgName=Msg  ProtocolMode=CAN  MsgIDType=Standard (11-bit identifier)  MsgIdentifier=4  MsgLength=8  SignalInfo={}  IDPort=off  TimestampPort=off  ErrorPort=off  RemotePort=off  LengthPort=off  StatusPort=off  BRSPort=off  ESIPort=off  DLCPort=off  ApplyMinMax=off
      settings: LibrarySourceBlock=stmutilitieslib/CAN FD Unpack  DataFormat=raw data
  CAN FD Unpack4 : canfdmsglib/CAN FD Unpack  MsgList=(none)  MsgName=Msg  ProtocolMode=CAN  MsgIDType=Standard (11-bit identifier)  MsgIdentifier=5  MsgLength=8  SignalInfo={}  IDPort=off  TimestampPort=off  ErrorPort=off  RemotePort=off  LengthPort=off  StatusPort=off  BRSPort=off  ESIPort=off  DLCPort=off  ApplyMinMax=off
      settings: LibrarySourceBlock=stmutilitieslib/CAN FD Unpack  DataFormat=raw data
  Data Type Conversion{1..5,7..14} (13 alike) : DataTypeConversion  OutDataTypeStr=boolean  SaturateOnIntegerOverflow=off  RndMeth=Floor
  Data Type Conversion{15..21} (7 alike) : DataTypeConversion  OutDataTypeStr=double  SaturateOnIntegerOverflow=off  RndMeth=Floor
  Data Type Conversion6 : DataTypeConversion  OutDataTypeStr=uint8  SaturateOnIntegerOverflow=off  RndMeth=Floor
  Extract Bits : simulink/Logic and Bit Operations/Extract Bits  bitsToExtract=Range of bits  numBits=8  bitIdxRange=[0]  outScalingMode=Treat bit field as an integer
  Extract Bits1 : simulink/Logic and Bit Operations/Extract Bits  bitsToExtract=Range of bits  numBits=8  bitIdxRange=[3]  outScalingMode=Treat bit field as an integer
  Extract Bits10 : simulink/Logic and Bit Operations/Extract Bits  bitsToExtract=Range of bits  numBits=8  bitIdxRange=[5]  outScalingMode=Treat bit field as an integer
  Extract Bits11 : simulink/Logic and Bit Operations/Extract Bits  bitsToExtract=Range of bits  numBits=8  bitIdxRange=[6]  outScalingMode=Treat bit field as an integer
  Extract Bits12 : simulink/Logic and Bit Operations/Extract Bits  bitsToExtract=Range of bits  numBits=8  bitIdxRange=[7]  outScalingMode=Treat bit field as an integer
  Extract Bits2 : simulink/Logic and Bit Operations/Extract Bits  bitsToExtract=Range of bits  numBits=8  bitIdxRange=[4]  outScalingMode=Treat bit field as an integer
  Extract Bits3 : simulink/Logic and Bit Operations/Extract Bits  bitsToExtract=Range of bits  numBits=8  bitIdxRange=[5]  outScalingMode=Treat bit field as an integer
  Extract Bits4 : simulink/Logic and Bit Operations/Extract Bits  bitsToExtract=Range of bits  numBits=8  bitIdxRange=[6]  outScalingMode=Treat bit field as an integer
  Extract Bits5 : simulink/Logic and Bit Operations/Extract Bits  bitsToExtract=Range of bits  numBits=8  bitIdxRange=[0]  outScalingMode=Treat bit field as an integer
  Extract Bits6 : simulink/Logic and Bit Operations/Extract Bits  bitsToExtract=Range of bits  numBits=8  bitIdxRange=[1]  outScalingMode=Treat bit field as an integer
  Extract Bits7 : simulink/Logic and Bit Operations/Extract Bits  bitsToExtract=Range of bits  numBits=8  bitIdxRange=[2]  outScalingMode=Treat bit field as an integer
  Extract Bits8 : simulink/Logic and Bit Operations/Extract Bits  bitsToExtract=Range of bits  numBits=8  bitIdxRange=[3]  outScalingMode=Treat bit field as an integer
  Extract Bits9 : simulink/Logic and Bit Operations/Extract Bits  bitsToExtract=Range of bits  numBits=8  bitIdxRange=[4]  outScalingMode=Treat bit field as an integer
  FDCAN Read1 : stm32blockslib/FDCAN Read  FDCANModule=FDCAN1  BlockMode=Receive  OperationReadMode=Data  OperationWriteMode=Data  ReadSource=FIFO 0  BufferNumber=0  OutputTypeReadMode=Packed  DataFormatWriteMode=Raw data  CANFrameType=CAN-FD  IdentifierTypeVia=Dialog  IdentifierType=Standard (11-bit identifier)  IdentifierVia=Inport  Identifier=100  DataLengthVia=Inport  DataLength=64  OutputIdType=off  IsBitRateSwitchingEnabled=off  TransmitRemoteFrame=off  OutputFrameType=off  OutputBRS=off  OutputRemoteFrame=off  OutputTxFifoLevel=off  OutputRxFifoLevel=off  OutputStatus=off  Timeout=0.001  SampleTime=-1
      settings: LibrarySourceBlock=stm32l5xxblockslib/FDCAN Read
  Selector : Selector  InputPortWidth=8  IndexOptions=Index vector (dialog)  Indices=[1 ]  OutputSizes=1
  Selector1 : Selector  InputPortWidth=8  IndexOptions=Index vector (dialog)  Indices=[2 ]  OutputSizes=1
  Selector{10..11,14..15} (4 alike) : Selector  InputPortWidth=8  IndexOptions=Index vector (dialog)  Indices=[5 ]  OutputSizes=1
  Selector12 : Selector  InputPortWidth=8  IndexOptions=Index vector (dialog)  Indices=[1 2 ]  OutputSizes=1
  Selector13 : Selector  InputPortWidth=8  IndexOptions=Index vector (dialog)  Indices=[3 4 ]  OutputSizes=1
  Selector2 : Selector  InputPortWidth=8  IndexOptions=Index vector (dialog)  Indices=[1 ]  OutputSizes=1
  Selector3 : Selector  InputPortWidth=8  IndexOptions=Index vector (dialog)  Indices=[2 ]  OutputSizes=1
  Selector4 : Selector  InputPortWidth=8  IndexOptions=Index vector (dialog)  Indices=[3 ]  OutputSizes=1
  Selector5 : Selector  InputPortWidth=8  IndexOptions=Index vector (dialog)  Indices=[4 ]  OutputSizes=1
  Selector6 : Selector  InputPortWidth=8  IndexOptions=Index vector (dialog)  Indices=[5 6 ]  OutputSizes=1
  Selector7 : Selector  InputPortWidth=8  IndexOptions=Index vector (dialog)  Indices=[7 8 ]  OutputSizes=1
  Selector8 : Selector  InputPortWidth=8  IndexOptions=Index vector (dialog)  Indices=[1 2 ]  OutputSizes=1
  Selector9 : Selector  InputPortWidth=8  IndexOptions=Index vector (dialog)  Indices=[3 4 ]  OutputSizes=1
  Subsystem : Subsystem
      mask Display: image('ALL Can.jpg');
  Terminator : Terminator
  Terminator1 : Terminator
  Terminator2 : Terminator
  Out1 : Outport
  Out2 : Outport  Port=2
  Out3 : Outport  Port=3
  Out4 : Outport  Port=4
  Out5 : Outport  Port=5
  Out6 : Outport  Port=6
  Out7 : Outport  Port=7
  Out8 : Outport  Port=8
  Out9 : Outport  Port=9
  Out10 : Outport  Port=10
  Out11 : Outport  Port=11
  Out12 : Outport  Port=12
  Out13 : Outport  Port=13
  Out14 : Outport  Port=14
  Out15 : Outport  Port=15
  Out16 : Outport  Port=16
  Out17 : Outport  Port=17
  Out18 : Outport  Port=18
  Out19 : Outport  Port=19
  Out20 : Outport  Port=20
  Out21 : Outport  Port=21
  Out22 : Outport  Port=22
  Out23 : Outport  Port=23
  Out24 : Outport  Port=24
  wires:
  CAN FD Unpack2/1 -> Selector1/1, Selector/1  "From Dash to VCU"
  FDCAN Read1/1 -> CAN FD Unpack1/1, CAN FD Unpack4/1, CAN FD Unpack3/1, CAN FD Unpack2/1
  Selector/1 -> Extract Bits4/1, Extract Bits3/1, Extract Bits2/1, Extract Bits1/1, Extract Bits/1  "Byte 0"
  Extract Bits/1 -> Data Type Conversion2/1
  Data Type Conversion2/1 -> Out1/1  "Boolean yes/no start button"
  Extract Bits1/1 -> Data Type Conversion1/1
  Data Type Conversion1/1 -> Out2/1  "SCin"
  Extract Bits2/1 -> Data Type Conversion3/1
  Data Type Conversion3/1 -> Out3/1  "SCEstop"
  Extract Bits3/1 -> Data Type Conversion4/1
  Data Type Conversion4/1 -> Out4/1  "SCIS"
  Extract Bits4/1 -> Data Type Conversion5/1
  Data Type Conversion5/1 -> Out5/1  "SCBOTS"
  Selector1/1 -> Data Type Conversion6/1  "Byte 0"
  Data Type Conversion6/1 -> Terminator/1  "PowerLimitPercentage"
  CAN FD Unpack1/1 -> Selector7/1, Selector6/1, Selector5/1, Selector4/1, Selector3/1, Selector2/1  "From Pedal Box to VCU"
  Data Type Conversion9/1 -> Out8/1  "SteeringFail"
  Extract Bits7/1 -> Data Type Conversion9/1
  Extract Bits6/1 -> Data Type Conversion7/1
  Extract Bits9/1 -> Data Type Conversion11/1
  Extract Bits5/1 -> Data Type Conversion8/1
  Extract Bits8/1 -> Data Type Conversion10/1
  Data Type Conversion7/1 -> Out7/1  "BSEFail"
  Data Type Conversion8/1 -> Out6/1  "APPSFail"
  Data Type Conversion10/1 -> Out9/1  "APPSMatch"
  Data Type Conversion11/1 -> Out10/1  "BrakesON"
  Extract Bits11/1 -> Data Type Conversion12/1
  Extract Bits12/1 -> Data Type Conversion13/1
  Data Type Conversion13/1 -> Out13/1  "BSEMatch"
  Selector2/1 -> Extract Bits12/1, Extract Bits11/1, Extract Bits10/1, Extract Bits9/1, Extract Bits8/1, Extract Bits7/1, Extract Bits6/1, Extract Bits5/1  "Byte 0"
  Data Type Conversion12/1 -> Out12/1  "SoftwareError"
  Data Type Conversion14/1 -> Out11/1  "SoftwareBSPD"
  Extract Bits10/1 -> Data Type Conversion14/1
  Selector3/1 -> Data Type Conversion15/1  "Byte 0"
  Data Type Conversion15/1 -> Out14/1  "APPS Percentage"
  Selector4/1 -> Data Type Conversion16/1  "Byte 0"
  Data Type Conversion16/1 -> Out15/1  "Brakes Percentage"
  Selector5/1 -> Data Type Conversion17/1  "Byte 0"
  Data Type Conversion17/1 -> Out16/1  "Steering Percentage"
  Selector6/1 -> Byte Unpack/1  "Byte 0"
  Byte Unpack/1 -> Out17/1  "Wheel Speed Front Left"
  Selector7/1 -> Byte Unpack1/1  "Byte 0"
  Byte Unpack1/1 -> Out18/1  "Wheel Speed Front Right"
  CAN FD Unpack3/1 -> Selector11/1, Selector10/1, Selector9/1, Selector8/1  "BMS1"
  Selector8/1 -> Byte Unpack2/1  "Byte 0"
  Byte Unpack2/1 -> Out19/1  "BMS Current Sensor"
  Selector9/1 -> Byte Unpack3/1  "Byte 0"
  Byte Unpack3/1 -> Out20/1  "BMS Voltage"
  Selector10/1 -> Data Type Conversion18/1  "Byte 0"
  Data Type Conversion18/1 -> Out21/1  "BMS SOC"
  Selector11/1 -> Data Type Conversion19/1  "Byte 0"
  Data Type Conversion19/1 -> Out22/1  "BMS Temprature"
  CAN FD Unpack4/1 -> Selector15/1, Selector14/1, Selector13/1, Selector12/1  "BMS2"
  Selector12/1 -> Byte Unpack4/1  "Byte 0"
  Byte Unpack4/1 -> Terminator1/1  "DCL"
  Selector13/1 -> Byte Unpack5/1  "Byte 0"
  Byte Unpack5/1 -> Terminator2/1  "CCL"
  Selector14/1 -> Data Type Conversion20/1  "Byte 0"
  Data Type Conversion20/1 -> Out23/1  "BMS_Max_Cell_Temp"
  Selector15/1 -> Data Type Conversion21/1  "Byte 0"
  Data Type Conversion21/1 -> Out24/1  "BMS_Max_Cell_Temp"
